simulink model "doubleIntegratorControlCons"  (R2015b)
settings: Solver=ode8  StartTime=0.0  StopTime=2  FixedStep=0.01  RelTol=1e-3
settings Model: Creator=E183308  LastModifiedBy=E183308

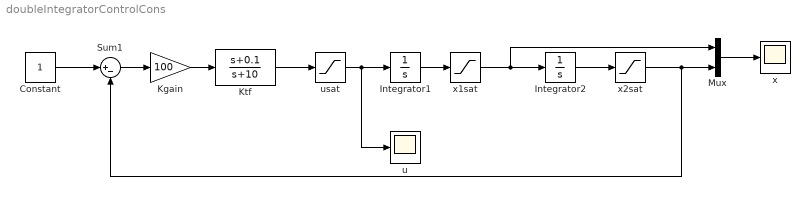
== system doubleIntegratorControlCons ==
  Constant : Constant
  Integrator1 : Integrator  UpperSaturationLimit=3  LowerSaturationLimit=-3
  Integrator2 : Integrator
  Kgain : Gain  Gain=100
  Ktf : TransferFcn  Numerator=[1 0.1]  Denominator=[1 10]
  Mux : Mux  Inputs=2
  Sum1 : Sum  Inputs=|+-
  u : Scope
  usat : Saturate  UpperLimit=3  LowerLimit=-3
  x : Scope
  x1sat : Saturate  UpperLimit=inf  LowerLimit=-inf
  x2sat : Saturate  UpperLimit=1  LowerLimit=-1
  wires:
  Integrator1/1 -> x1sat/1
  Integrator2/1 -> x2sat/1
  Constant/1 -> Sum1/1
  Ktf/1 -> usat/1
  Kgain/1 -> Ktf/1
  Sum1/1 -> Kgain/1
  Mux/1 -> x/1
  x1sat/1 -> Mux/1, Integrator2/1
  x2sat/1 -> Mux/2, Sum1/2
  usat/1 -> u/1, Integrator1/1
